simulink model "four_channel_bilateral_teleoperation"  (R2020b)
settings: Solver=ode45  StartTime=0.0  StopTime=10  FixedStep=Ts  MinStep=1e-5  RelTol=1e-5
undefined symbols (not defined in the file): A, Be, Bh_i, Bm, Bs, Dh, Dm, Ds, Fc, Fip, Jh_i, Ke, Kh, Kh_i, Km, Ks, Mm, Ms, Ts, xe
libraries: simulink x6, cstblocks x5
settings Model: Creator=simon  LastModifiedBy=SimoneCremasco
settings SolverCC: AlgebraicLoopSolver=LineSearch

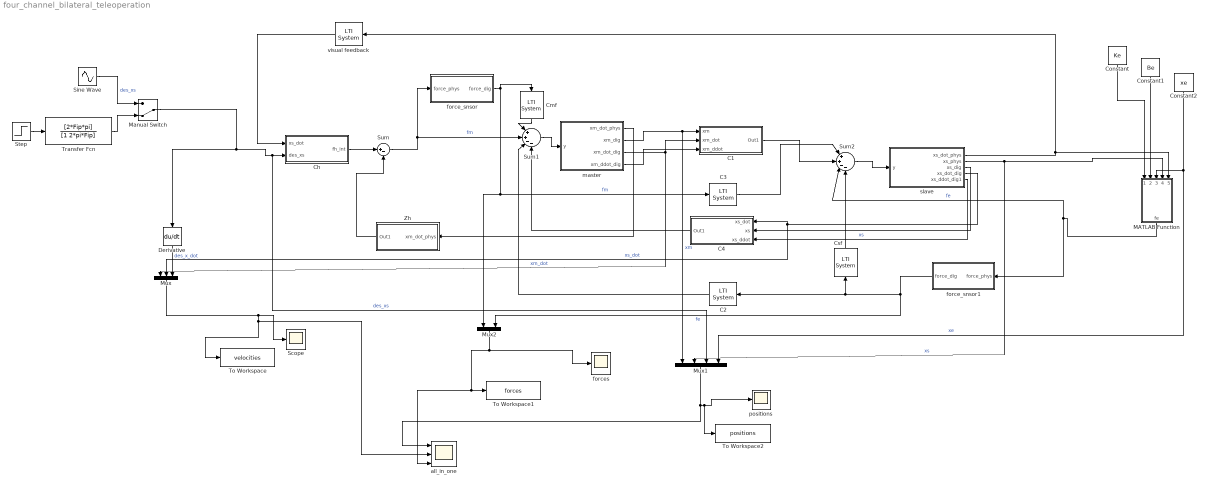
== system four_channel_bilateral_teleoperation ==
  C1 : Subsystem
  C2 : cstblocks/LTI System  sys=C2  IC=[]
  C3 : cstblocks/LTI System  sys=C3  IC=[]
  C4 : Subsystem
  Ch : Subsystem
  Cmf : cstblocks/LTI System  sys=Cmf  IC=[]
  Constant : Constant  Value=Ke
  Constant1 : Constant  Value=Be
  Constant2 : Constant  Value=xe
  Csf : cstblocks/LTI System  sys=Csf  IC=[]
  Derivative : Derivative
  MATLAB Function : MATLAB Function  TreatAsAtomicUnit=on
  Manual Switch : ManualSwitch  CurrentSetting=0
  Mux : Mux  Inputs=3
  Mux1 : Mux
  Mux2 : Mux  Inputs=2
  Scope : Scope
  Sine Wave : Sin  Amplitude=A  Frequency=2*pi*Fc  SampleTime=0
  Step : Step  SampleTime=0
  Sum : Sum  Inputs=|+-
  Sum1 : Sum  Inputs=|++--
  Sum2 : Sum  Inputs=|++--
  To Workspace : ToWorkspace  VariableName=velocities  SaveFormat=Timeseries  SampleTime=-1
  To Workspace1 : ToWorkspace  VariableName=forces  SaveFormat=Timeseries  SampleTime=-1
  To Workspace2 : ToWorkspace  VariableName=positions  SaveFormat=Timeseries  SampleTime=-1
  Transfer Fcn : TransferFcn  Numerator=[2*Fip*pi]  Denominator=[1 2*pi*Fip]
  Zh : Subsystem
  all_in_one : Scope  NumInputPorts=3
  force_snsor : Subsystem
  force_snsor1 : Subsystem
  forces : Scope
  master : Subsystem
  positions : Scope
  slave : Subsystem
  visual feedback : cstblocks/LTI System  sys=1  IC=[]
  wires:
  Zh/1(Out1) -> Sum/2
  Sum1/1 -> master/1(y)
  C4/1(Out1) -> Sum1/4
  C2/1 -> Sum1/3
  C3/1 -> Sum2/1
  C1/1(Out1) -> Sum2/2
  Sum2/1 -> slave/1(y)
  MATLAB Function/1(fe) -> Sum2/3, force_snsor1/1(force_phys)  "fe"
  Constant2/1 -> Mux1/4, MATLAB Function/3(xe)  "xe"
  Constant1/1 -> MATLAB Function/2(Be)
  Constant/1 -> MATLAB Function/1(Ke)
  Sum/1 -> force_snsor/1(force_phys), Sum1/2  "fm"
  Cmf/1 -> Sum1/1
  Csf/1 -> Sum2/4
  visual feedback/1 -> Ch/1(xs_dot)
  Ch/1(fh_int) -> Sum/1
  Manual Switch/1 -> Mux1/3, Ch/2(des_xs), Derivative/1  "des_xs"
  force_snsor/1(force_dig) -> Cmf/1, Mux2/1, C3/1  "fm"
  force_snsor1/1(force_dig) -> C2/1, Csf/1, Mux2/2  "fe"
  Derivative/1 -> Mux/3  "des_x_dot"
  Mux2/1 -> all_in_one/3, To Workspace1/1, forces/1
  Mux/1 -> To Workspace/1, all_in_one/2, Scope/1
  master/2(xm_dig) -> C1/1(xm), Mux1/1  "xm"
  master/3(xm_dot_dig) -> Mux/1, C1/2(xm_dot)  "xm_dot"
  slave/3(xs_dig) -> C4/2(xs)  "xs"
  slave/4(xs_dot_dig) -> Mux/2, C4/1(xs_dot)  "xs_dot"
  master/1(xm_dot_phys) -> Zh/1(xm_dot_phys)
  slave/1(xs_dot_phys) -> visual feedback/1, MATLAB Function/5(dxs)
  slave/2(xs_phys) -> Mux1/2, MATLAB Function/4(xs)  "xs"
  master/4(xm_ddot_dig) -> C1/3(xm_ddot)
  slave/5(xs_ddot_dig1) -> C4/3(xs_ddot)
  Mux1/1 -> all_in_one/1, To Workspace2/1, positions/1
  Sine Wave/1 -> Manual Switch/1  "des_xs"
  Step/1 -> Transfer Fcn/1
  Transfer Fcn/1 -> Manual Switch/2

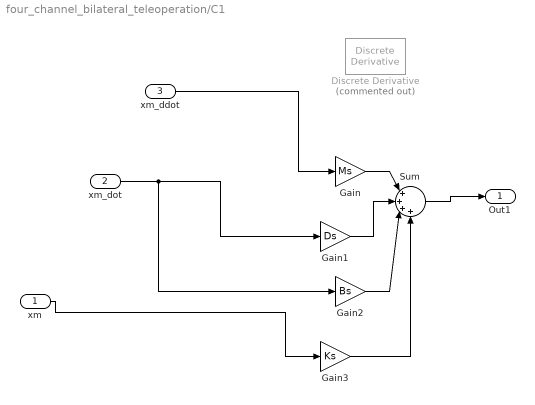
== system four_channel_bilateral_teleoperation/C1 ==
  xm : Inport
  xm_dot : Inport  Port=2
  xm_ddot : Inport  Port=3
  Discrete Derivative : simulink/Discrete/Discrete Derivative  Commented=on  gainval=1.0  ICPrevScaledInput=0.0  OutMin=[]  OutMax=[]  OutDataType=fixdt(1, 16)  OutScaling=2^-10  DoSatur=off
  Gain : Gain  Gain=Ms
  Gain1 : Gain  Gain=Ds
  Gain2 : Gain  Gain=Bs
  Gain3 : Gain  Gain=Ks
  Sum : Sum  Inputs=|++++
  Out1 : Outport
  wires:
  xm_dot/1 -> Gain2/1, Gain1/1
  xm_ddot/1 -> Gain/1
  Gain/1 -> Sum/1
  Gain1/1 -> Sum/2
  xm/1 -> Gain3/1
  Gain2/1 -> Sum/3
  Gain3/1 -> Sum/4
  Sum/1 -> Out1/1

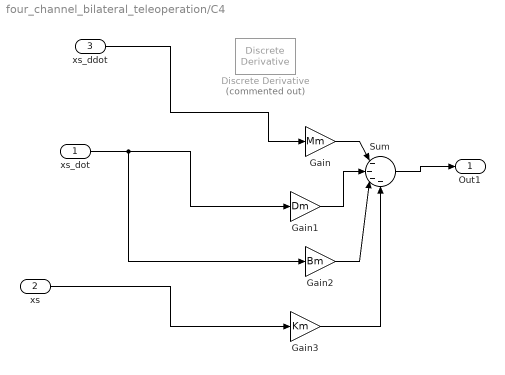
== system four_channel_bilateral_teleoperation/C4 ==
  xs_dot : Inport
  xs : Inport  Port=2
  xs_ddot : Inport  Port=3
  Discrete Derivative : simulink/Discrete/Discrete Derivative  Commented=on  gainval=1.0  ICPrevScaledInput=0.0  OutMin=[]  OutMax=[]  OutDataType=fixdt(1, 16)  OutScaling=2^-10  DoSatur=off
  Gain : Gain  Gain=Mm
  Gain1 : Gain  Gain=Dm
  Gain2 : Gain  Gain=Bm
  Gain3 : Gain  Gain=Km
  Sum : Sum  Inputs=|----
  Out1 : Outport
  wires:
  xs_dot/1 -> Gain2/1, Gain1/1
  xs_ddot/1 -> Gain/1
  Gain/1 -> Sum/1
  Gain1/1 -> Sum/2
  xs/1 -> Gain3/1
  Gain2/1 -> Sum/3
  Gain3/1 -> Sum/4
  Sum/1 -> Out1/1

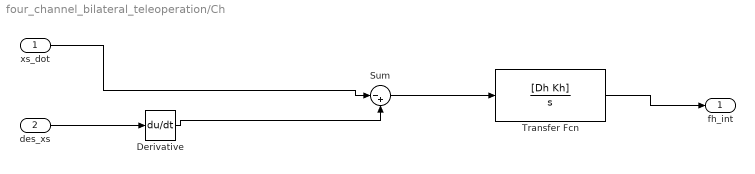
== system four_channel_bilateral_teleoperation/Ch ==
  xs_dot : Inport
  des_xs : Inport  Port=2
  Derivative : Derivative
  Sum : Sum  Inputs=|-+
  Transfer Fcn : TransferFcn  Numerator=[Dh Kh]  Denominator=[1 0]
  fh_int : Outport
  wires:
  xs_dot/1 -> Sum/1
  des_xs/1 -> Derivative/1
  Derivative/1 -> Sum/2
  Sum/1 -> Transfer Fcn/1
  Transfer Fcn/1 -> fh_int/1

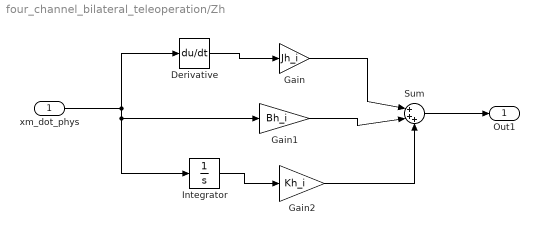
== system four_channel_bilateral_teleoperation/Zh ==
  xm_dot_phys : Inport
  Derivative : Derivative
  Gain : Gain  Gain=Jh_i
  Gain1 : Gain  Gain=Bh_i
  Gain2 : Gain  Gain=Kh_i
  Integrator : Integrator
  Sum : Sum  Inputs=|+++
  Out1 : Outport
  wires:
  Derivative/1 -> Gain/1
  Integrator/1 -> Gain2/1
  xm_dot_phys/1 -> Integrator/1, Gain1/1, Derivative/1
  Gain/1 -> Sum/1
  Gain1/1 -> Sum/2
  Gain2/1 -> Sum/3
  Sum/1 -> Out1/1

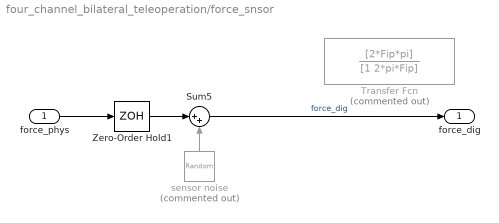
== system four_channel_bilateral_teleoperation/force_snsor ==
  force_phys : Inport
  Sum5 : Sum  Inputs=|++
  Transfer Fcn : TransferFcn  Commented=on  Numerator=[2*Fip*pi]  Denominator=[1 2*pi*Fip]
  Zero-Order Hold1 : ZeroOrderHold  SampleTime=Ts
  sensor noise : RandomNumber  Commented=on  Variance=0.0000001  SampleTime=Ts
  force_dig : Outport
  wires:
  Sum5/1 -> force_dig/1  "force_dig"
  Zero-Order Hold1/1 -> Sum5/1
  sensor noise/1 -> Sum5/2
  force_phys/1 -> Zero-Order Hold1/1

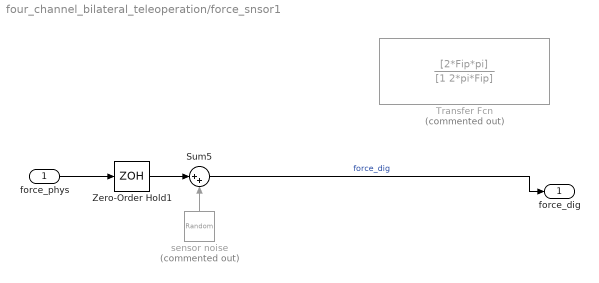
== system four_channel_bilateral_teleoperation/force_snsor1 ==
  force_phys : Inport
  Sum5 : Sum  Inputs=|++
  Transfer Fcn : TransferFcn  Commented=on  Numerator=[2*Fip*pi]  Denominator=[1 2*pi*Fip]
  Zero-Order Hold1 : ZeroOrderHold  SampleTime=Ts
  sensor noise : RandomNumber  Commented=on  Variance=0.0000001  SampleTime=Ts
  force_dig : Outport
  wires:
  Sum5/1 -> force_dig/1  "force_dig"
  Zero-Order Hold1/1 -> Sum5/1
  sensor noise/1 -> Sum5/2
  force_phys/1 -> Zero-Order Hold1/1

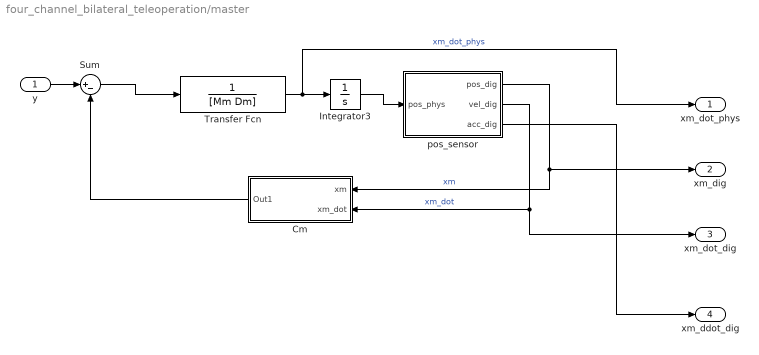
== system four_channel_bilateral_teleoperation/master ==
  y : Inport
  Cm : Subsystem
  Integrator3 : Integrator
  Sum : Sum  Inputs=|+-
  Transfer Fcn : TransferFcn  Denominator=[Mm Dm]
  pos_sensor : Subsystem
  xm_dot_phys : Outport
  xm_dig : Outport  Port=2
  xm_dot_dig : Outport  Port=3
  xm_ddot_dig : Outport  Port=4
  wires:
  pos_sensor/2(vel_dig) -> xm_dot_dig/1, Cm/2(xm_dot)  "xm_dot"
  pos_sensor/1(pos_dig) -> xm_dig/1, Cm/1(xm)  "xm"
  y/1 -> Sum/1
  Sum/1 -> Transfer Fcn/1
  Cm/1(Out1) -> Sum/2
  Transfer Fcn/1 -> xm_dot_phys/1, Integrator3/1  "xm_dot_phys"
  Integrator3/1 -> pos_sensor/1(pos_phys)
  pos_sensor/3(acc_dig) -> xm_ddot_dig/1

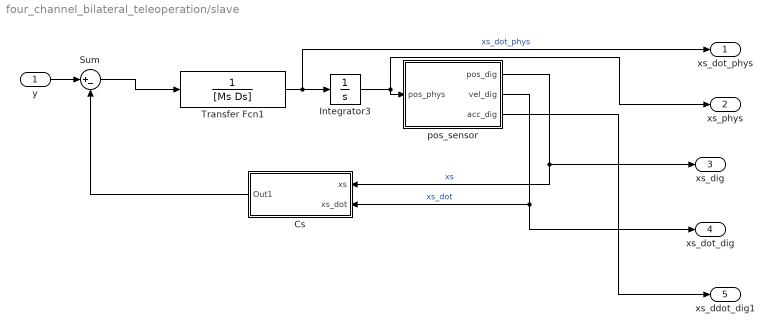
== system four_channel_bilateral_teleoperation/slave ==
  y : Inport
  Cs : Subsystem
  Integrator3 : Integrator
  Sum : Sum  Inputs=|+-
  Transfer Fcn1 : TransferFcn  Denominator=[Ms Ds]
  pos_sensor : Subsystem
  xs_dot_phys : Outport
  xs_phys : Outport  Port=2
  xs_dig : Outport  Port=3
  xs_dot_dig : Outport  Port=4
  xs_ddot_dig1 : Outport  Port=5
  wires:
  pos_sensor/2(vel_dig) -> Cs/2(xs_dot), xs_dot_dig/1  "xs_dot"
  pos_sensor/1(pos_dig) -> Cs/1(xs), xs_dig/1  "xs"
  y/1 -> Sum/1
  Sum/1 -> Transfer Fcn1/1
  Cs/1(Out1) -> Sum/2
  Transfer Fcn1/1 -> xs_dot_phys/1, Integrator3/1  "xs_dot_phys"
  Integrator3/1 -> xs_phys/1, pos_sensor/1(pos_phys)
  pos_sensor/3(acc_dig) -> xs_ddot_dig1/1

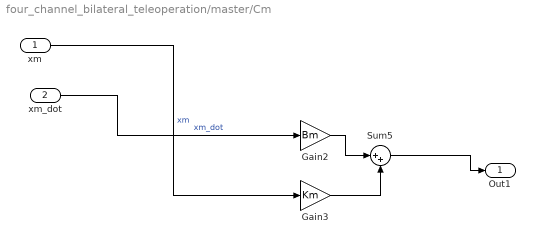
== system four_channel_bilateral_teleoperation/master/Cm ==
  xm : Inport
  xm_dot : Inport  Port=2
  Gain2 : Gain  Gain=Bm
  Gain3 : Gain  Gain=Km
  Sum5 : Sum  Inputs=|++
  Out1 : Outport
  wires:
  xm/1 -> Gain3/1  "xm"
  Gain2/1 -> Sum5/1
  xm_dot/1 -> Gain2/1  "xm_dot"
  Gain3/1 -> Sum5/2
  Sum5/1 -> Out1/1

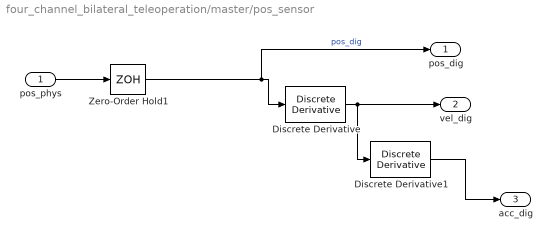
== system four_channel_bilateral_teleoperation/master/pos_sensor ==
  pos_phys : Inport
  Discrete Derivative : simulink/Discrete/Discrete Derivative  gainval=1.0  ICPrevScaledInput=0.0  OutMin=[]  OutMax=[]  OutDataType=fixdt(1, 16)  OutScaling=2^-10  DoSatur=off
  Discrete Derivative1 : simulink/Discrete/Discrete Derivative  gainval=1.0  ICPrevScaledInput=0.0  OutMin=[]  OutMax=[]  OutDataType=fixdt(1, 16)  OutScaling=2^-10  DoSatur=off
  Zero-Order Hold1 : ZeroOrderHold  SampleTime=Ts
  pos_dig : Outport
  vel_dig : Outport  Port=2
  acc_dig : Outport  Port=3
  wires:
  pos_phys/1 -> Zero-Order Hold1/1
  Zero-Order Hold1/1 -> pos_dig/1, Discrete Derivative/1  "pos_dig"
  Discrete Derivative/1 -> Discrete Derivative1/1, vel_dig/1
  Discrete Derivative1/1 -> acc_dig/1

== system four_channel_bilateral_teleoperation/slave/Cs ==
  xs : Inport
  xs_dot : Inport  Port=2
  Gain : Gain  Gain=Bs
  Gain1 : Gain  Gain=Ks
  Sum4 : Sum  Inputs=|++
  Out1 : Outport
  wires:
  Gain1/1 -> Sum4/2
  Sum4/1 -> Out1/1
  xs_dot/1 -> Gain/1  "xs_dot"
  Gain/1 -> Sum4/1
  xs/1 -> Gain1/1  "xs"

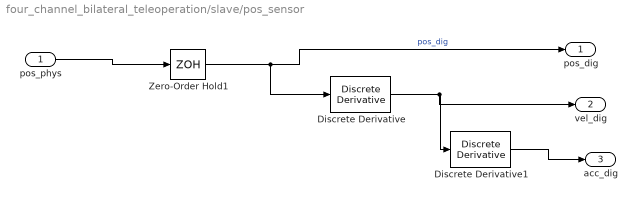
== system four_channel_bilateral_teleoperation/slave/pos_sensor ==
  pos_phys : Inport
  Discrete Derivative : simulink/Discrete/Discrete Derivative  gainval=1.0  ICPrevScaledInput=0.0  OutMin=[]  OutMax=[]  OutDataType=fixdt(1, 16)  OutScaling=2^-10  DoSatur=off
  Discrete Derivative1 : simulink/Discrete/Discrete Derivative  gainval=1.0  ICPrevScaledInput=0.0  OutMin=[]  OutMax=[]  OutDataType=fixdt(1, 16)  OutScaling=2^-10  DoSatur=off
  Zero-Order Hold1 : ZeroOrderHold  SampleTime=Ts
  pos_dig : Outport
  vel_dig : Outport  Port=2
  acc_dig : Outport  Port=3
  wires:
  Zero-Order Hold1/1 -> Discrete Derivative/1, pos_dig/1  "pos_dig"
  pos_phys/1 -> Zero-Order Hold1/1
  Discrete Derivative/1 -> vel_dig/1, Discrete Derivative1/1
  Discrete Derivative1/1 -> acc_dig/1

== matlab function four_channel_bilateral_teleoperation/MATLAB Function ==
  data: Ke input; fe output; Be input; xe input; xs input; dxs input
function fe = env(Ke, Be, xe, xs, dxs)
    if xs > xe
        fe = Ke*(xs-xe)+Be*max(dxs, 0);
    else
        fe = 0;
    end
